simulink model "problem1"  (Simulink 7.7)
settings: Solver=ode45  StartTime=0.0  StopTime=100.0  RelTol=1e-3
libraries: simulink x1
settings Model: Creator=Ed  LastModifiedBy=Ed

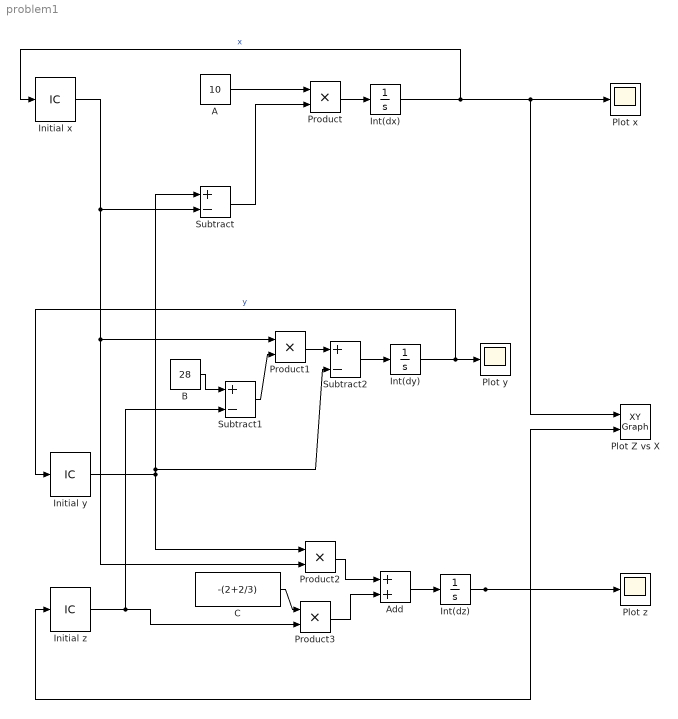
== system problem1 ==
  A : Constant  Value=10
  Add : Sum
  B : Constant  Value=28
  C : Constant  Value=-(2+2/3)
  Initial x : InitialCondition
  Initial y : InitialCondition
  Initial z : InitialCondition
  Int(dx) : Integrator
  Int(dy) : Integrator
  Int(dz) : Integrator
  Plot Z vs X : simulink/Sinks/XY Graph  SystemSampleTime=-1  xmin=-1  xmax=50  ymin=-1  ymax=50  st=-1
  Plot x : Scope
  Plot y : Scope
  Plot z : Scope
      settings: SaveName=ScopeData2
  Product{,1..3} (4 alike) : Product  RndMeth=Zero
  Subtract : Sum  Inputs=+-
  Subtract1 : Sum  Inputs=+-
  Subtract2 : Sum  Inputs=+-
  wires:
  Int(dx)/1 -> Initial x/1, Plot x/1, Plot Z vs X/1  "x"
  Product/1 -> Int(dx)/1
  Subtract/1 -> Product/2
  Int(dy)/1 -> Initial y/1, Plot y/1  "y"
  Subtract1/1 -> Product1/2
  Subtract2/1 -> Int(dy)/1
  Product1/1 -> Subtract2/1
  Product2/1 -> Add/1
  Product3/1 -> Add/2
  Add/1 -> Int(dz)/1
  A/1 -> Product/1
  B/1 -> Subtract1/1
  C/1 -> Product3/1
  Initial x/1 -> Subtract/2, Product1/1, Product2/2
  Initial y/1 -> Product2/1, Subtract/1, Subtract2/2
  Initial z/1 -> Subtract1/2, Product3/2
  Int(dz)/1 -> Initial z/1, Plot z/1, Plot Z vs X/2
